simulink model "fuzzy_pid"  (R2019a)
settings: Solver=VariableStepAuto  StartTime=0.0  StopTime=10.0  RelTol=1e-3
libraries: simulink x1
settings Model: Creator=intel  LastModifiedBy=intel
settings SolverCC: MaxConsecutiveMinStep=3

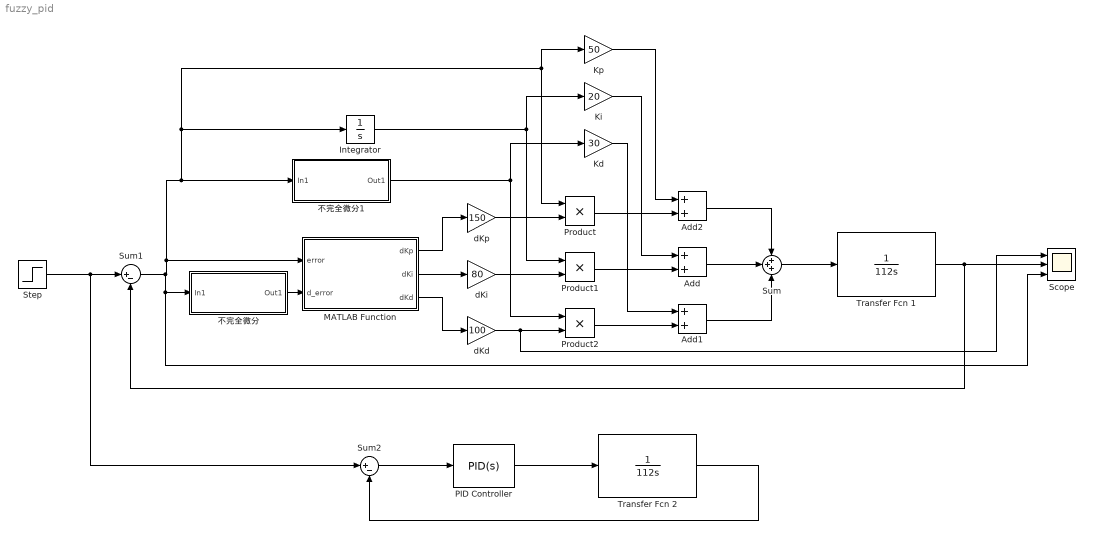
== system fuzzy_pid ==
  Add : Sum
  Add1 : Sum
  Add2 : Sum
  Integrator : Integrator
  Kd : Gain  Gain=30
  Ki : Gain  Gain=20
  Kp : Gain  Gain=50
  MATLAB Function : MATLAB Function  TreatAsAtomicUnit=on
  PID Controller : simulink/Continuous/PID Controller  Controller=PID  Form=Parallel  TimeDomain=Continuous-time  SampleTime=-1  IntegratorMethod=Forward Euler  FilterMethod=Forward Euler  ControllerParametersSource=internal  P=200  I=80  D=50  UseFilter=on  N=100  TunerSelectOption=Transfer Function Based (PID Tuner App)  InitialConditionSource=internal  InitialConditionForIntegrator=0  InitialConditionForFilter=0  DifferentiatorICPrevScaledInput=0  ExternalReset=none  TrackingMode=off  Kt=1  LimitOutput=off  UpperSaturationLimit=inf  LowerSaturationLimit=-inf  LinearizeAsGain=on  AntiWindupMode=none  Kb=1  POutMin=[]  POutMax=[]  IOutMin=[]  IOutMax=[]  DOutMin=[]  DOutMax=[]  NOutMin=[]  NOutMax=[]  SumOutMin=[]  SumOutMax=[]  SaturationOutMin=[]  SaturationOutMax=[]  PParamMin=[]  PParamMax=[]  IParamMin=[]  IParamMax=[]  DParamMin=[]  DParamMax=[]  NParamMin=[]  NParamMax=[]  KbParamMin=[]  KbParamMax=[]  KtParamMin=[]  KtParamMax=[]  KbOutMin=[]  KbOutMax=[]  KtOutMin=[]  KtOutMax=[]  IntegratorOutMin=[]  IntegratorOutMax=[]  FilterOutMin=[]  FilterOutMax=[]  SumI1OutMin=[]  SumI1OutMax=[]  SumI2OutMin=[]  SumI2OutMax=[]  SumI3OutMin=[]  SumI3OutMax=[]  SumI4OutMin=[]  SumI4OutMax=[]  SumDOutMin=[]  SumDOutMax=[]  DifferentiatorOutMin=[]  DifferentiatorOutMax=[]  FilterDiffOutCoefMin=[]  FilterDiffOutCoefMax=[]  ReciprocalOutMin=[]  ReciprocalOutMax=[]  SumDenOutMin=[]  SumDenOutMax=[]  SumNumOutMin=[]  SumNumOutMax=[]  DivideOutMin=[]  DivideOutMax=[]  IntegratorContinuousStateAttributes=''  IntegratorStateMustResolveToSignalObject=off  IntegratorRTWStateStorageClass=Auto  FilterContinuousStateAttributes=''  FilterStateMustResolveToSignalObject=off  FilterRTWStateStorageClass=Auto  ParallelPVariant=InternalParameters  IdealPVariant=Disabled  IVariant=InternalParameters  DVariant=InternalParameters  IntegratorVariant=Continuous  SatVariant=Disabled  AWVariant=Passthrough  PCopyVariant=Disabled  TRVariant=Disabled  FdbkBlocksVariant=Forward  IdealPFdbkVariant=Disabled  SatFdbkVariant=Disabled  DerivativeFilterVariant=ContFilter  NVariant=InternalParameters  NCopyVariant=Disabled  FilterICVariant=InternalICsFilter  IntegratorICVariant=InternalICs  ExternalResetVariant=Disabled  TRSumVariant=Passthrough  SumFdbkVariant=Disabled  SumVariant=Sum_PID
  Product : Product
  Product1 : Product
  Product2 : Product
  Scope : Scope  NumInputPorts=3
  Step : Step  SampleTime=0
  Sum : Sum  Inputs=+++
  Sum1 : Sum  Inputs=|+-
  Sum2 : Sum  Inputs=|+-
  Transfer Fcn 1 : TransferFcn  Denominator=[112 0]
  Transfer Fcn 2 : TransferFcn  Denominator=[112 0]
  dKd : Gain  Gain=100
  dKi : Gain  Gain=80
  dKp : Gain  Gain=150
  不完全微分 : Subsystem
  不完全微分1 : Subsystem
  wires:
  Transfer Fcn 1/1 -> Scope/2, Sum1/2
  Step/1 -> Sum1/1, Sum2/1
  Sum1/1 -> Scope/3, 不完全微分/1(In1), MATLAB Function/1(error), 不完全微分1/1(In1), Integrator/1, Kp/1, Product/1
  MATLAB Function/1(dKp) -> dKp/1
  MATLAB Function/2(dKi) -> dKi/1
  MATLAB Function/3(dKd) -> dKd/1
  dKp/1 -> Product/2
  dKi/1 -> Product1/2
  dKd/1 -> Scope/1, Product2/2
  不完全微分1/1(Out1) -> Product2/1, Kd/1
  Integrator/1 -> Product1/1, Ki/1
  Product/1 -> Add2/2
  Product1/1 -> Add/2
  Product2/1 -> Add1/2
  Kd/1 -> Add1/1
  Ki/1 -> Add/1
  Kp/1 -> Add2/1
  Add/1 -> Sum/2
  Add2/1 -> Sum/1
  Add1/1 -> Sum/3
  Sum/1 -> Transfer Fcn 1/1
  PID Controller/1 -> Transfer Fcn 2/1
  Sum2/1 -> PID Controller/1
  Transfer Fcn 2/1 -> Sum2/2
  不完全微分/1(Out1) -> MATLAB Function/2(d_error)

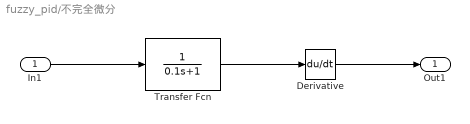
== system fuzzy_pid/不完全微分 ==
  In1 : Inport
  Derivative : Derivative
  Transfer Fcn : TransferFcn  Denominator=[0.1 1]
  Out1 : Outport
  wires:
  In1/1 -> Transfer Fcn/1
  Transfer Fcn/1 -> Derivative/1
  Derivative/1 -> Out1/1

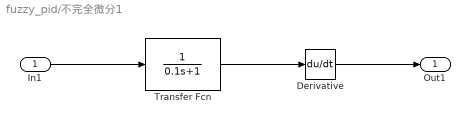
== system fuzzy_pid/不完全微分1 ==
  In1 : Inport
  Derivative : Derivative
  Transfer Fcn : TransferFcn  Denominator=[0.1 1]
  Out1 : Outport
  wires:
  In1/1 -> Transfer Fcn/1
  Transfer Fcn/1 -> Derivative/1
  Derivative/1 -> Out1/1

== matlab function fuzzy_pid/MATLAB Function ==
  data: error input; dKp output; d_error input; dKi output; dKd output
function [dKp,dKi,dKd] = FuzzyCal(error,d_error)
    [dKp,dKi,dKd]=FuzzyComputation(error,d_error);
end
